simulink model "Diskretni_TG_test"  (R2021b)
settings: Solver=VariableStepAuto  StartTime=0.0  StopTime=0.05  RelTol=1e-3
values from neighbouring files (symbols this model uses):
  Gp = tf(K,conv([T1 1],[T2 1]))    [TG_dc_discrete_motor.m]
  Gr = minreal(1/Gp*Gm/(1-Gm))    [TG_dc_discrete_motor.m]
  Grd = minreal(1/Gpd*Gmz/(1-Gmz))    [TG_dc_discrete_motor.m]
  T = 2e-3    (= 0.002)    [TG_dc_discrete_motor.m]
settings Model: Creator=jmatusko  LastModifiedBy=jmatusko

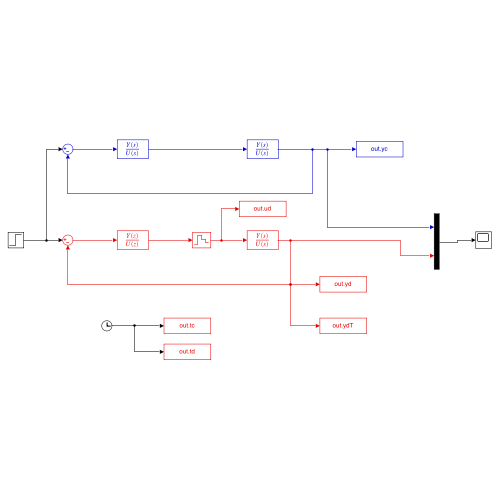
[thumbnail: Simulink's stored preview of the top-level diagram]
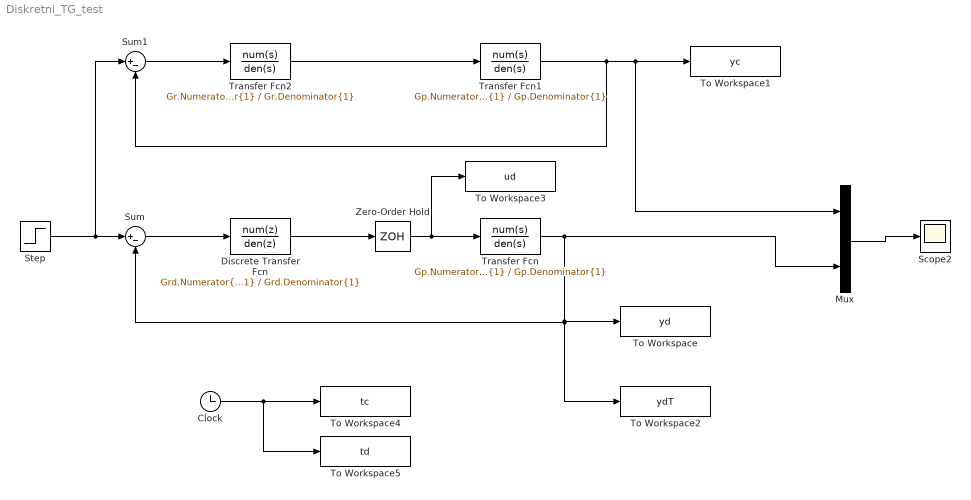
== system Diskretni_TG_test ==
  Clock : Clock
  Discrete Transfer Fcn : DiscreteTransferFcn  Numerator=Grd.Numerator{1}  Denominator=Grd.Denominator{1}  SampleTime=T
  Mux : Mux  Inputs=2
  Scope2 : Scope
  Step : Step  Time=0  SampleTime=0
  Sum : Sum  Inputs=|+-
  Sum1 : Sum  Inputs=|+-
  To Workspace : ToWorkspace  VariableName=yd  SampleTime=T/10
  To Workspace1 : ToWorkspace  VariableName=yc  SampleTime=T/10
  To Workspace2 : ToWorkspace  VariableName=ydT  SampleTime=T
  To Workspace3 : ToWorkspace  VariableName=ud  SampleTime=T/10
  To Workspace4 : ToWorkspace  VariableName=tc  SampleTime=T/10
  To Workspace5 : ToWorkspace  VariableName=td  SampleTime=T
  Transfer Fcn : TransferFcn  Numerator=Gp.Numerator{1}  Denominator=Gp.Denominator{1}
  Transfer Fcn1 : TransferFcn  Numerator=Gp.Numerator{1}  Denominator=Gp.Denominator{1}
  Transfer Fcn2 : TransferFcn  Numerator=Gr.Numerator{1}  Denominator=Gr.Denominator{1}
  Zero-Order Hold : ZeroOrderHold  SampleTime=T
  wires:
  Zero-Order Hold/1 -> To Workspace3/1, Transfer Fcn/1
  Discrete Transfer Fcn/1 -> Zero-Order Hold/1
  Sum/1 -> Discrete Transfer Fcn/1
  Transfer Fcn/1 -> To Workspace2/1, Sum/2, To Workspace/1, Mux/2
  Step/1 -> Sum/1, Sum1/1
  Transfer Fcn1/1 -> Sum1/2, Mux/1, To Workspace1/1
  Sum1/1 -> Transfer Fcn2/1
  Transfer Fcn2/1 -> Transfer Fcn1/1
  Mux/1 -> Scope2/1
  Clock/1 -> To Workspace5/1, To Workspace4/1
